simulink model "platooning_with_csma_simulink"  (R2017b)
settings: Solver=VariableStepAuto  StartTime=0.0  StopTime=t_end  FixedStep=timestep  RelTol=1e-3
model workspace (MAT data in the model file):
  t_0 = 0
values from neighbouring files (symbols this model uses):
  a_max = 1.0 * a_factor    (= 1)    [platooning_with_csma.m]
  a_min = -0.5 * a_factor    (= -0.5)    [platooning_with_csma.m]
  follower_1 = car    [platooning_with_csma.m]
  follower_2 = car    [platooning_with_csma.m]
  leader = car    [platooning_with_csma.m]
  N = 1000    [platooning_with_csma.m]
  remove_trigger_time = 0.01    [platooning_with_csma.m]
  timestep = 1e-3    (= 0.001)    [platooning_with_csma.m]
libraries: truetime x6, dspstat3 x2, dspindex x2, simulink x1
settings Model: Creator=s132652  LastModifiedBy=s132652
settings CodeAppCC: StateflowObjectComments=on

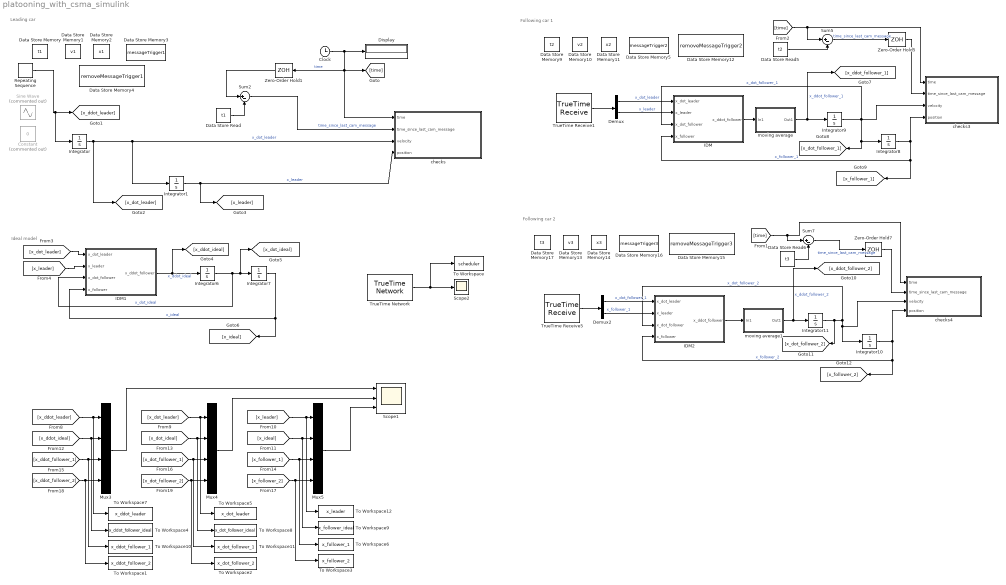
== system platooning_with_csma_simulink ==
  note: Leading car
  note: Ideal model
  note: Following car 1
  note: Following car 2
  Clock : Clock
  Constant : Constant  Commented=on  Value=0
  Data Store Memory : DataStoreMemory  DataStoreName=t1  ReadBeforeWriteMsg=warning  WriteAfterWriteMsg=warning  WriteAfterReadMsg=warning  ShowAdditionalParam=off
  Data Store Memory1 : DataStoreMemory  DataStoreName=v1  ReadBeforeWriteMsg=warning  WriteAfterWriteMsg=warning  WriteAfterReadMsg=warning  InitialValue=leader.v0  ShowAdditionalParam=off
  Data Store Memory10 : DataStoreMemory  DataStoreName=v2  ReadBeforeWriteMsg=warning  WriteAfterWriteMsg=warning  WriteAfterReadMsg=warning  InitialValue=follower_1.v0  ShowAdditionalParam=off
  Data Store Memory11 : DataStoreMemory  DataStoreName=x2  ReadBeforeWriteMsg=warning  WriteAfterWriteMsg=warning  WriteAfterReadMsg=warning  InitialValue=follower_1.x0  ShowAdditionalParam=off
  Data Store Memory12 : DataStoreMemory  DataStoreName=removeMessageTrigger2  ReadBeforeWriteMsg=warning  WriteAfterWriteMsg=warning  WriteAfterReadMsg=warning  ShowAdditionalParam=off
  Data Store Memory13 : DataStoreMemory  DataStoreName=v3  ReadBeforeWriteMsg=warning  WriteAfterWriteMsg=warning  WriteAfterReadMsg=warning  InitialValue=follower_2.v0  ShowAdditionalParam=off
  Data Store Memory14 : DataStoreMemory  DataStoreName=x3  ReadBeforeWriteMsg=warning  WriteAfterWriteMsg=warning  WriteAfterReadMsg=warning  InitialValue=follower_2.x0  ShowAdditionalParam=off
  Data Store Memory15 : DataStoreMemory  DataStoreName=removeMessageTrigger3  ReadBeforeWriteMsg=warning  WriteAfterWriteMsg=warning  WriteAfterReadMsg=warning  ShowAdditionalParam=off
  Data Store Memory16 : DataStoreMemory  DataStoreName=messageTrigger3  ReadBeforeWriteMsg=warning  WriteAfterWriteMsg=warning  WriteAfterReadMsg=warning  ShowAdditionalParam=off
  Data Store Memory17 : DataStoreMemory  DataStoreName=t3  ReadBeforeWriteMsg=warning  WriteAfterWriteMsg=warning  WriteAfterReadMsg=warning  ShowAdditionalParam=off
  Data Store Memory2 : DataStoreMemory  DataStoreName=x1  ReadBeforeWriteMsg=warning  WriteAfterWriteMsg=warning  WriteAfterReadMsg=warning  InitialValue=leader.x0  ShowAdditionalParam=off
  Data Store Memory3 : DataStoreMemory  DataStoreName=messageTrigger1  ReadBeforeWriteMsg=warning  WriteAfterWriteMsg=warning  WriteAfterReadMsg=warning  ShowAdditionalParam=off
  Data Store Memory4 : DataStoreMemory  DataStoreName=removeMessageTrigger1  ReadBeforeWriteMsg=warning  WriteAfterWriteMsg=warning  WriteAfterReadMsg=warning  ShowAdditionalParam=off
  Data Store Memory5 : DataStoreMemory  DataStoreName=messageTrigger2  ReadBeforeWriteMsg=warning  WriteAfterWriteMsg=warning  WriteAfterReadMsg=warning  ShowAdditionalParam=off
  Data Store Memory9 : DataStoreMemory  DataStoreName=t2  ReadBeforeWriteMsg=warning  WriteAfterWriteMsg=warning  WriteAfterReadMsg=warning  ShowAdditionalParam=off
  Data Store Read : DataStoreRead  DataStoreName=t1
  Data Store Read5 : DataStoreRead  DataStoreName=t2
  Data Store Read6 : DataStoreRead  DataStoreName=t3
  Demux : Demux  Outputs=2
  Demux2 : Demux  Outputs=2
  Display : Display
  IDM : Subsystem
  IDM1 : Subsystem
  IDM2 : Subsystem
  Integrator : Integrator  InitialCondition=leader.v0
  Integrator1 : Integrator  InitialCondition=leader.x0
  Integrator10 : Integrator  InitialCondition=follower_2.x0
  Integrator11 : Integrator  InitialCondition=follower_2.v0
  Integrator6 : Integrator  InitialCondition=follower_1.v0
  Integrator7 : Integrator  InitialCondition=follower_1.x0
  Integrator8 : Integrator  InitialCondition=follower_1.x0
  Integrator9 : Integrator  InitialCondition=follower_1.v0
  Mux3 : Mux
  Mux4 : Mux
  Mux5 : Mux
  Repeating Sequence : simulink/Sources/Repeating Sequence  rep_seq_t=[0 5 10 15 20 25 30 35 40 45 50 55 60 65 70]  rep_seq_y=[0 0 0 0 0 a_max a_max 0 0 0 a_min a_min 0 0 0]
  Scope1 : Scope  NumInputPorts=3
  Scope2 : Scope
  Sine Wave : Sin  Commented=on  Frequency=2*pi/10  SampleTime=0
  Sum2 : Sum  Inputs=|+-
  Sum5 : Sum  Inputs=|+-
  Sum7 : Sum  Inputs=|+-
  To Workspace : ToWorkspace  VariableName=scheduler  SaveFormat=Timeseries  SampleTime=-1
  To Workspace1 : ToWorkspace  VariableName=x_ddot_follower_2  SaveFormat=Timeseries  SampleTime=-1
  To Workspace10 : ToWorkspace  VariableName=x_ddot_follower_1  SaveFormat=Timeseries  SampleTime=-1
  To Workspace11 : ToWorkspace  VariableName=x_dot_follower_1  SaveFormat=Timeseries  SampleTime=-1
  To Workspace12 : ToWorkspace  VariableName=x_leader  SaveFormat=Timeseries  SampleTime=-1
  To Workspace2 : ToWorkspace  VariableName=x_dot_follower_2  SaveFormat=Timeseries  SampleTime=-1
  To Workspace3 : ToWorkspace  VariableName=x_follower_2  SaveFormat=Timeseries  SampleTime=-1
  To Workspace4 : ToWorkspace  VariableName=x_ddot_follower_ideal  SaveFormat=Timeseries  SampleTime=-1
  To Workspace5 : ToWorkspace  VariableName=x_dot_leader  SaveFormat=Timeseries  SampleTime=-1
  To Workspace6 : ToWorkspace  VariableName=x_follower_1  SaveFormat=Timeseries  SampleTime=-1
  To Workspace7 : ToWorkspace  VariableName=x_ddot_leader  SaveFormat=Timeseries  SampleTime=-1
  To Workspace8 : ToWorkspace  VariableName=x_dot_follower_ideal  SaveFormat=Timeseries  SampleTime=-1
  To Workspace9 : ToWorkspace  VariableName=x_follower_ideal  SaveFormat=Timeseries  SampleTime=-1
  TrueTime Network : truetime/TrueTime Network  nwtype=CSMA/AMP (CAN)  nwnbr=1  nnodes=3  rate=data_rate  minsize=512  lossprob=0  seed=0  bandwidths=[0.5 0.5]  slotsize=512  schedule=[1 1 2]  memsize=80000  buftype=Common buffer  overflow=Retransmit  dynSchedule=0  miniSlotSize=0  NIT=0  QSortMode=FIFO  sync=0  irtSchedule=0  nrtLength=0  nodeGraph=0  scheduleoutput=on
  TrueTime Receive1 : truetime/TrueTime Receive  nwnbr=1  receiver=1  outdim=2  triggeroutput=off  senderoutput=off  lengthoutput=off  priorityoutput=off  timestampoutput=off  signalpoweroutput=off  msgIDoutput=off
  TrueTime Receive5 : truetime/TrueTime Receive  nwnbr=1  receiver=2  outdim=2  triggeroutput=off  senderoutput=off  lengthoutput=off  priorityoutput=off  timestampoutput=off  signalpoweroutput=off  msgIDoutput=off
  Zero-Order Hold1 : ZeroOrderHold  SampleTime=timestep
  Zero-Order Hold5 : ZeroOrderHold  SampleTime=timestep
  Zero-Order Hold7 : ZeroOrderHold  SampleTime=timestep
  checks : Subsystem
  checks3 : Subsystem
  checks4 : Subsystem
  moving average : Subsystem
  moving average1 : Subsystem
  wires:
  TrueTime Network/1 -> To Workspace/1, Scope2/1
  Sum2/1 -> checks/2(time_since_last_cam_message)  "time_since_last_cam_message"
  Data Store Read/1 -> Sum2/2
  Integrator6/1 -> IDM1/3(x_dot_follower), [x_dot_ideal], Integrator7/1  "x_dot_ideal"
  Integrator/1 -> [x_dot_leader], Integrator1/1, checks/3(velocity)  "x_dot_leader"
  IDM1/1(x_ddot_follower) -> [x_ddot_ideal], Integrator6/1  "x_ddot_ideal"
  Integrator7/1 -> [x_ideal], IDM1/4(x_follower)  "x_ideal"
  Integrator1/1 -> [x_leader], checks/4(position)  "x_leader"
  moving average/1(Out1) -> [x_ddot_follower_1], Integrator9/1  "x_ddot_follower_1"
  Integrator8/1 -> [x_follower_1], IDM/4(x_follower), checks3/4(position)  "x_follower_1"
  Integrator9/1 -> [x_dot_follower_1], Integrator8/1, checks3/3(velocity), IDM/3(x_dot_follower)  "x_dot_follower_1"
  IDM/1(x_ddot_follower) -> moving average/1(In1)
  TrueTime Receive1/1 -> Demux/1
  Zero-Order Hold5/1 -> checks3/2(time_since_last_cam_message)
  Data Store Read5/1 -> Sum5/2
  Sum5/1 -> Zero-Order Hold5/1  "time_since_last_cam_message"
  Clock/1 -> checks/1(time), [time], Zero-Order Hold1/1, Display/1  "time"
  Zero-Order Hold7/1 -> checks4/2(time_since_last_cam_message)
  moving average1/1(Out1) -> [x_ddot_follower_2], Integrator11/1  "x_ddot_follower_2"
  Sum7/1 -> Zero-Order Hold7/1  "time_since_last_cam_message"
  TrueTime Receive5/1 -> Demux2/1
  Data Store Read6/1 -> Sum7/2
  Integrator10/1 -> IDM2/4(x_follower), [x_follower_2], checks4/4(position)  "x_follower_2"
  Integrator11/1 -> [x_dot_follower_2], IDM2/3(x_dot_follower), checks4/3(velocity), Integrator10/1  "x_dot_follower_2"
  IDM2/1(x_ddot_follower) -> moving average1/1(In1)
  [time] -> checks4/1(time), Sum7/1
  [time] -> Sum5/1, checks3/1(time)
  [x_dot_leader] -> IDM1/1(x_dot_leader)
  [x_leader] -> IDM1/2(x_leader)
  [x_ddot_leader] -> To Workspace7/1, Mux3/1
  [x_ddot_ideal] -> To Workspace4/1, Mux3/2
  [x_ddot_follower_1] -> To Workspace10/1, Mux3/3
  [x_ddot_follower_2] -> To Workspace1/1, Mux3/4
  [x_dot_leader] -> To Workspace5/1, Mux4/1
  [x_dot_ideal] -> To Workspace8/1, Mux4/2
  [x_dot_follower_1] -> To Workspace11/1, Mux4/3
  [x_dot_follower_2] -> To Workspace2/1, Mux4/4
  [x_follower_2] -> To Workspace3/1, Mux5/4
  [x_follower_1] -> To Workspace6/1, Mux5/3
  [x_ideal] -> To Workspace9/1, Mux5/2
  [x_leader] -> To Workspace12/1, Mux5/1
  Mux3/1 -> Scope1/1
  Mux4/1 -> Scope1/2
  Mux5/1 -> Scope1/3
  Zero-Order Hold1/1 -> Sum2/1
  Demux/2 -> IDM/2(x_leader)  "x_leader"
  Demux/1 -> IDM/1(x_dot_leader)  "x_dot_leader"
  Demux2/1 -> IDM2/1(x_dot_leader)  "x_dot_follower_1"
  Demux2/2 -> IDM2/2(x_leader)  "x_follower_1"
  Repeating Sequence/1 -> Integrator/1, [x_ddot_leader]

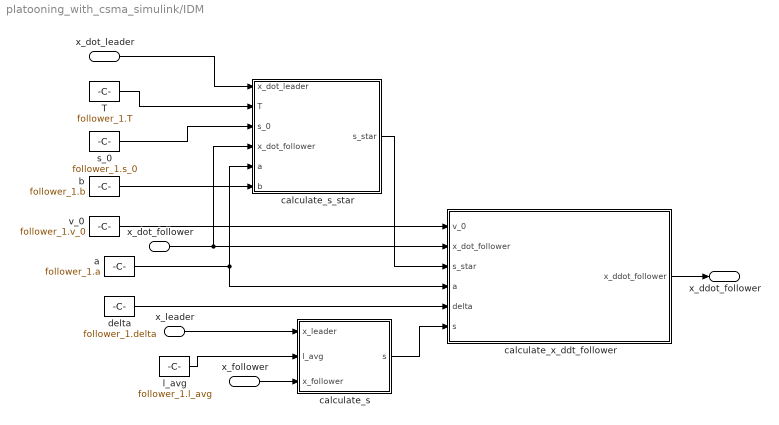
== system platooning_with_csma_simulink/IDM ==
  x_dot_leader : Inport
  x_leader : Inport  Port=2
  x_dot_follower : Inport  Port=3
  x_follower : Inport  Port=4
  T : Constant  Value=follower_1.T
  a : Constant  Value=follower_1.a
  b : Constant  Value=follower_1.b
  calculate_s : Subsystem
  calculate_s_star : Subsystem
  calculate_x_ddt_follower : Subsystem
  delta : Constant  Value=follower_1.delta
  l_avg : Constant  Value=follower_1.l_avg
  s_0 : Constant  Value=follower_1.s_0
  v_0 : Constant  Value=follower_1.v_0
  x_ddot_follower : Outport
  wires:
  v_0/1 -> calculate_x_ddt_follower/1(v_0)
  T/1 -> calculate_s_star/2(T)
  s_0/1 -> calculate_s_star/3(s_0)
  calculate_x_ddt_follower/1(x_ddot_follower) -> x_ddot_follower/1
  b/1 -> calculate_s_star/6(b)
  l_avg/1 -> calculate_s/2(l_avg)
  calculate_s/1(s) -> calculate_x_ddt_follower/6(s)
  delta/1 -> calculate_x_ddt_follower/5(delta)
  calculate_s_star/1(s_star) -> calculate_x_ddt_follower/3(s_star)
  x_follower/1 -> calculate_s/3(x_follower)
  x_dot_leader/1 -> calculate_s_star/1(x_dot_leader)
  x_leader/1 -> calculate_s/1(x_leader)
  x_dot_follower/1 -> calculate_s_star/4(x_dot_follower), calculate_x_ddt_follower/2(x_dot_follower)
  a/1 -> calculate_x_ddt_follower/4(a), calculate_s_star/5(a)

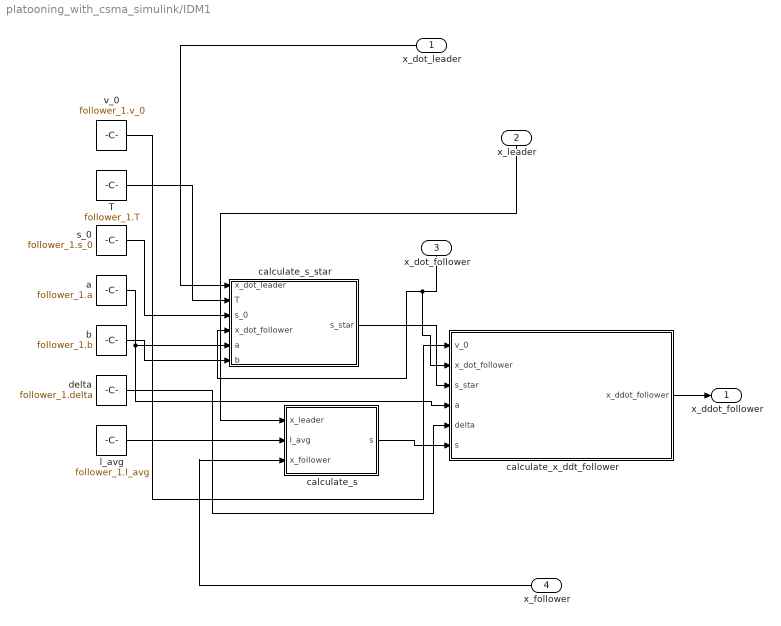
== system platooning_with_csma_simulink/IDM1 ==
  x_dot_leader : Inport
  x_leader : Inport  Port=2
  x_dot_follower : Inport  Port=3
  x_follower : Inport  Port=4
  T : Constant  Value=follower_1.T
  a : Constant  Value=follower_1.a
  b : Constant  Value=follower_1.b
  calculate_s : Subsystem
  calculate_s_star : Subsystem
  calculate_x_ddt_follower : Subsystem
  delta : Constant  Value=follower_1.delta
  l_avg : Constant  Value=follower_1.l_avg
  "s_0 " : Constant  Value=follower_1.s_0
  v_0 : Constant  Value=follower_1.v_0
  x_ddot_follower : Outport
  wires:
  a/1 -> calculate_x_ddt_follower/4(a), calculate_s_star/5(a)
  v_0/1 -> calculate_x_ddt_follower/1(v_0)
  T/1 -> calculate_s_star/2(T)
  "s_0 "/1 -> calculate_s_star/3(s_0)
  calculate_x_ddt_follower/1(x_ddot_follower) -> x_ddot_follower/1
  b/1 -> calculate_s_star/6(b)
  l_avg/1 -> calculate_s/2(l_avg)
  calculate_s/1(s) -> calculate_x_ddt_follower/6(s)
  delta/1 -> calculate_x_ddt_follower/5(delta)
  calculate_s_star/1(s_star) -> calculate_x_ddt_follower/3(s_star)
  x_follower/1 -> calculate_s/3(x_follower)
  x_dot_follower/1 -> calculate_x_ddt_follower/2(x_dot_follower), calculate_s_star/4(x_dot_follower)
  x_dot_leader/1 -> calculate_s_star/1(x_dot_leader)
  x_leader/1 -> calculate_s/1(x_leader)

== system platooning_with_csma_simulink/IDM2 ==
  x_dot_leader : Inport
  x_leader : Inport  Port=2
  x_dot_follower : Inport  Port=3
  x_follower : Inport  Port=4
  T : Constant  Value=follower_2.T
  a : Constant  Value=follower_2.a
  b : Constant  Value=follower_2.b
  calculate_s : Subsystem
  calculate_s_star : Subsystem
  calculate_x_ddt_follower : Subsystem
  delta : Constant  Value=follower_2.delta
  l_avg : Constant  Value=follower_2.l_avg
  s_0 : Constant  Value=follower_2.s_0
  v_0 : Constant  Value=follower_2.v_0
  x_ddot_follower : Outport
  wires:
  v_0/1 -> calculate_x_ddt_follower/1(v_0)
  T/1 -> calculate_s_star/2(T)
  s_0/1 -> calculate_s_star/3(s_0)
  calculate_x_ddt_follower/1(x_ddot_follower) -> x_ddot_follower/1
  b/1 -> calculate_s_star/6(b)
  l_avg/1 -> calculate_s/2(l_avg)
  calculate_s/1(s) -> calculate_x_ddt_follower/6(s)
  delta/1 -> calculate_x_ddt_follower/5(delta)
  calculate_s_star/1(s_star) -> calculate_x_ddt_follower/3(s_star)
  x_follower/1 -> calculate_s/3(x_follower)
  x_dot_leader/1 -> calculate_s_star/1(x_dot_leader)
  x_leader/1 -> calculate_s/1(x_leader)
  x_dot_follower/1 -> calculate_s_star/4(x_dot_follower), calculate_x_ddt_follower/2(x_dot_follower)
  a/1 -> calculate_x_ddt_follower/4(a), calculate_s_star/5(a)

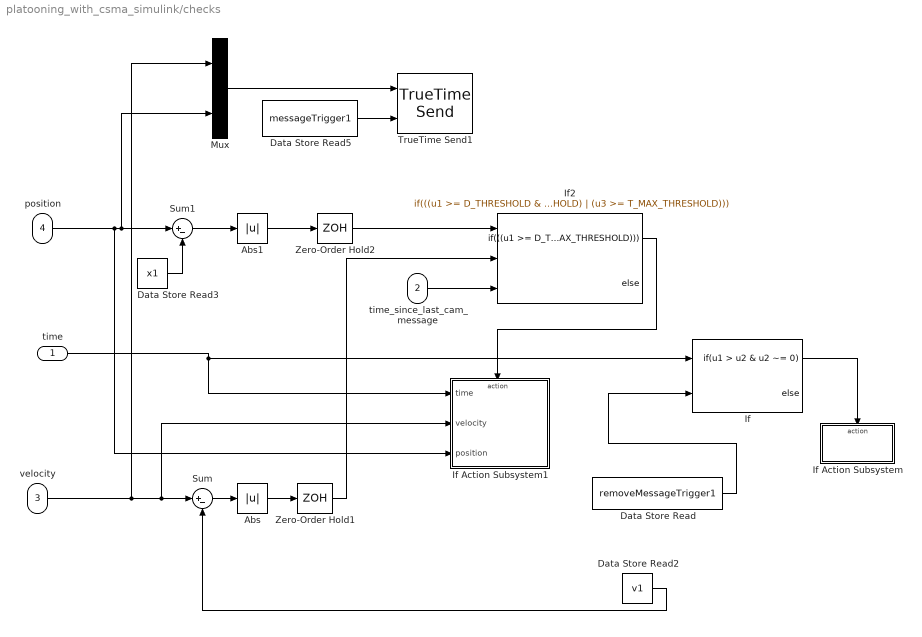
== system platooning_with_csma_simulink/checks ==
  time : Inport
  time_since_last_cam_message : Inport  Port=2
  velocity : Inport  Port=3
  position : Inport  Port=4
  Abs : Abs
  Abs1 : Abs
  Data Store Read : DataStoreRead  DataStoreName=removeMessageTrigger1
  Data Store Read2 : DataStoreRead  DataStoreName=v1
  Data Store Read3 : DataStoreRead  DataStoreName=x1
  Data Store Read5 : DataStoreRead  DataStoreName=messageTrigger1
  If : If  NumInputs=2  IfExpression=u1 > u2 & u2 ~= 0
  If Action Subsystem : Subsystem  TreatAsAtomicUnit=on
  If Action Subsystem1 : Subsystem  TreatAsAtomicUnit=on
  If2 : If  NumInputs=3  IfExpression=((u1 >= D_THRESHOLD & u3 >= T_MIN_THRESHOLD) | (u2 >= S_THRESHOLD & u3 >= T_MIN_THRESHOLD) | (u3 >= T_MAX_THRESHOLD))
  Mux : Mux  Inputs=2
  Sum : Sum  Inputs=|+-
  Sum1 : Sum  Inputs=|+-
  TrueTime Send1 : truetime/TrueTime Send  trigger=rising  nwnbr=1  sender=1  indim=2  recsource=internal  receiver=1  lengthsource=internal  length=data_length  priosource=internal  prio=1  msgIDsource=internal  msgID=0  dynamicSegment=dynamic
  Zero-Order Hold1 : ZeroOrderHold  SampleTime=timestep
  Zero-Order Hold2 : ZeroOrderHold  SampleTime=timestep
  wires:
  Data Store Read3/1 -> Sum1/2
  Sum1/1 -> Abs1/1
  Abs1/1 -> Zero-Order Hold2/1
  Zero-Order Hold2/1 -> If2/1
  time/1 -> If/1, If Action Subsystem1/1(time)
  position/1 -> Mux/2, Sum1/1, If Action Subsystem1/3(position)
  If2/1 -> If Action Subsystem1/Action
  Abs/1 -> Zero-Order Hold1/1
  Sum/1 -> Abs/1
  Data Store Read2/1 -> Sum/2
  velocity/1 -> Mux/1, If Action Subsystem1/2(velocity), Sum/1
  time_since_last_cam_message/1 -> If2/3
  Zero-Order Hold1/1 -> If2/2
  Mux/1 -> TrueTime Send1/1
  Data Store Read5/1 -> TrueTime Send1/2
  If/1 -> If Action Subsystem/Action
  Data Store Read/1 -> If/2

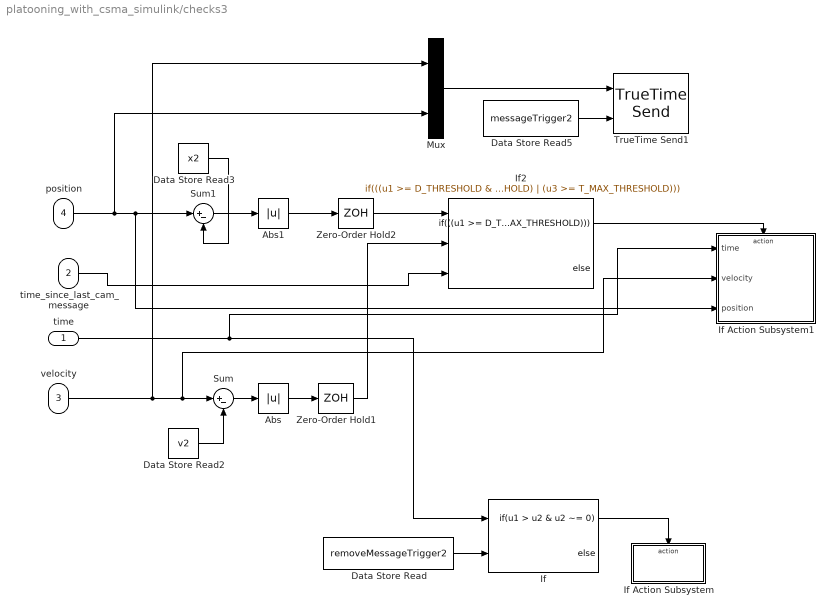
== system platooning_with_csma_simulink/checks3 ==
  time : Inport
  time_since_last_cam_message : Inport  Port=2
  velocity : Inport  Port=3
  position : Inport  Port=4
  Abs : Abs
  Abs1 : Abs
  Data Store Read : DataStoreRead  DataStoreName=removeMessageTrigger2
  Data Store Read2 : DataStoreRead  DataStoreName=v2
  Data Store Read3 : DataStoreRead  DataStoreName=x2
  Data Store Read5 : DataStoreRead  DataStoreName=messageTrigger2
  If : If  NumInputs=2  IfExpression=u1 > u2 & u2 ~= 0
  If Action Subsystem : Subsystem  TreatAsAtomicUnit=on
  If Action Subsystem1 : Subsystem  TreatAsAtomicUnit=on
  If2 : If  NumInputs=3  IfExpression=((u1 >= D_THRESHOLD & u3 >= T_MIN_THRESHOLD) | (u2 >= S_THRESHOLD & u3 >= T_MIN_THRESHOLD) | (u3 >= T_MAX_THRESHOLD))
  Mux : Mux  Inputs=2
  Sum : Sum  Inputs=|+-
  Sum1 : Sum  Inputs=|+-
  TrueTime Send1 : truetime/TrueTime Send  trigger=rising  nwnbr=1  sender=2  indim=2  recsource=internal  receiver=2  lengthsource=internal  length=data_length  priosource=internal  prio=1  msgIDsource=internal  msgID=0  dynamicSegment=dynamic
  Zero-Order Hold1 : ZeroOrderHold  SampleTime=timestep
  Zero-Order Hold2 : ZeroOrderHold  SampleTime=timestep
  wires:
  Data Store Read3/1 -> Sum1/2
  Sum1/1 -> Abs1/1
  Abs1/1 -> Zero-Order Hold2/1
  Zero-Order Hold2/1 -> If2/1
  time/1 -> If/1, If Action Subsystem1/1(time)
  position/1 -> Mux/2, If Action Subsystem1/3(position), Sum1/1
  If2/1 -> If Action Subsystem1/Action
  Abs/1 -> Zero-Order Hold1/1
  Sum/1 -> Abs/1
  Data Store Read2/1 -> Sum/2
  velocity/1 -> If Action Subsystem1/2(velocity), Sum/1, Mux/1
  time_since_last_cam_message/1 -> If2/3
  Zero-Order Hold1/1 -> If2/2
  Mux/1 -> TrueTime Send1/1
  Data Store Read5/1 -> TrueTime Send1/2
  If/1 -> If Action Subsystem/Action
  Data Store Read/1 -> If/2

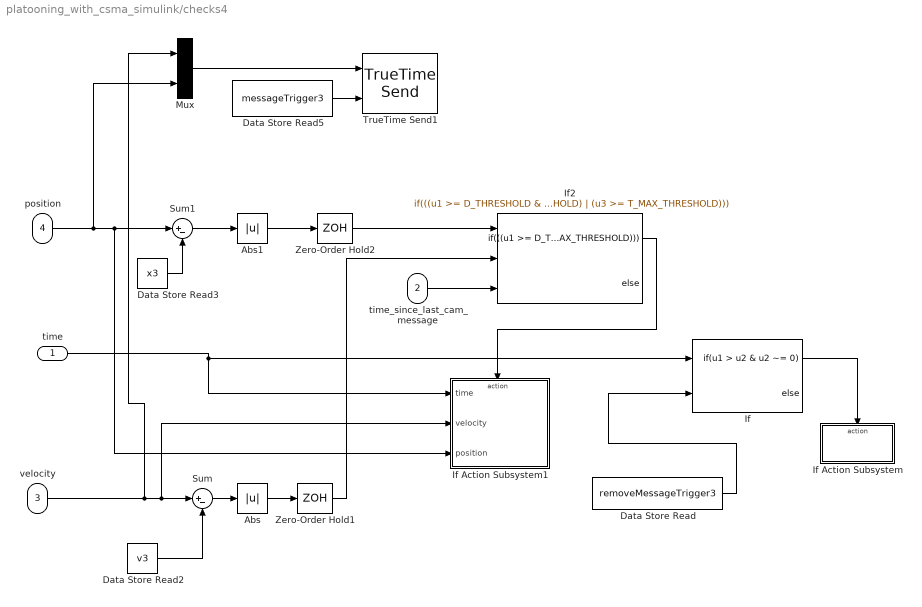
== system platooning_with_csma_simulink/checks4 ==
  time : Inport
  time_since_last_cam_message : Inport  Port=2
  velocity : Inport  Port=3
  position : Inport  Port=4
  Abs : Abs
  Abs1 : Abs
  Data Store Read : DataStoreRead  DataStoreName=removeMessageTrigger3
  Data Store Read2 : DataStoreRead  DataStoreName=v3
  Data Store Read3 : DataStoreRead  DataStoreName=x3
  Data Store Read5 : DataStoreRead  DataStoreName=messageTrigger3
  If : If  NumInputs=2  IfExpression=u1 > u2 & u2 ~= 0
  If Action Subsystem : Subsystem  TreatAsAtomicUnit=on
  If Action Subsystem1 : Subsystem  TreatAsAtomicUnit=on
  If2 : If  NumInputs=3  IfExpression=((u1 >= D_THRESHOLD & u3 >= T_MIN_THRESHOLD) | (u2 >= S_THRESHOLD & u3 >= T_MIN_THRESHOLD) | (u3 >= T_MAX_THRESHOLD))
  Mux : Mux  Inputs=2
  Sum : Sum  Inputs=|+-
  Sum1 : Sum  Inputs=|+-
  TrueTime Send1 : truetime/TrueTime Send  trigger=rising  nwnbr=1  sender=3  indim=2  recsource=internal  receiver=3  lengthsource=internal  length=data_length  priosource=internal  prio=1  msgIDsource=internal  msgID=0  dynamicSegment=dynamic
  Zero-Order Hold1 : ZeroOrderHold  SampleTime=-1
  Zero-Order Hold2 : ZeroOrderHold  SampleTime=timestep
  wires:
  Data Store Read3/1 -> Sum1/2
  Sum1/1 -> Abs1/1
  Abs1/1 -> Zero-Order Hold2/1
  Zero-Order Hold2/1 -> If2/1
  time/1 -> If/1, If Action Subsystem1/1(time)
  position/1 -> Mux/2, Sum1/1, If Action Subsystem1/3(position)
  If2/1 -> If Action Subsystem1/Action
  Abs/1 -> Zero-Order Hold1/1
  Sum/1 -> Abs/1
  Data Store Read2/1 -> Sum/2
  velocity/1 -> Mux/1, If Action Subsystem1/2(velocity), Sum/1
  time_since_last_cam_message/1 -> If2/3
  Zero-Order Hold1/1 -> If2/2
  Mux/1 -> TrueTime Send1/1
  Data Store Read5/1 -> TrueTime Send1/2
  If/1 -> If Action Subsystem/Action
  Data Store Read/1 -> If/2

== system platooning_with_csma_simulink/moving average ==
  note: moving average
  In1 : Inport
  IC : InitialCondition  Value=zeros(N,1)
  Mean : dspstat3/Mean  run=off  reset_popup=None  InputProcessing=Columns as channels (frame based)  directionMode=Each column  dimension=1  roiEnable=off  roiType=Rectangles  roiPortion=Entire ROI  roiOutput=Individual statistics for each ROI  roiFlag=off  outputDataTypeStr=Inherit: Same as accumulator  outputLastDataTypeStr=Inherit: Same as accumulator  outputMin=[]  outputMax=[]  roundingMode=Floor  overflowMode=off
  Memory : Memory
  Mux : Mux  Inputs=2
  Variable Selector : dspindex/Variable Selector  NumInputs=1  rowsOrCols=Rows  IdxMode=Fixed  Elements=1:N-1  ZerOneIdxMode=One-based  errmode=Clip Index  FillMode=on  FillValues=0
  Out1 : Outport
  wires:
  In1/1 -> Mux/1
  Mux/1 -> Mean/1, Memory/1
  Memory/1 -> IC/1
  IC/1 -> Variable Selector/1
  Mean/1 -> Out1/1
  Variable Selector/1 -> Mux/2

== system platooning_with_csma_simulink/moving average1 ==
  note: moving average
  In1 : Inport
  IC : InitialCondition  Value=zeros(N,1)
  Mean : dspstat3/Mean  run=off  reset_popup=None  InputProcessing=Columns as channels (frame based)  directionMode=Each column  dimension=1  roiEnable=off  roiType=Rectangles  roiPortion=Entire ROI  roiOutput=Individual statistics for each ROI  roiFlag=off  outputDataTypeStr=Inherit: Same as accumulator  outputLastDataTypeStr=Inherit: Same as accumulator  outputMin=[]  outputMax=[]  roundingMode=Floor  overflowMode=off
  Memory : Memory
  Mux : Mux  Inputs=2
  Variable Selector : dspindex/Variable Selector  NumInputs=1  rowsOrCols=Rows  IdxMode=Fixed  Elements=1:N-1  ZerOneIdxMode=One-based  errmode=Clip Index  FillMode=on  FillValues=0
  Out1 : Outport
  wires:
  In1/1 -> Mux/1
  Mux/1 -> Mean/1, Memory/1
  Memory/1 -> IC/1
  IC/1 -> Variable Selector/1
  Mean/1 -> Out1/1
  Variable Selector/1 -> Mux/2

== system platooning_with_csma_simulink/IDM/calculate_s ==
  x_leader : Inport
  l_avg : Inport  Port=2
  x_follower : Inport  Port=3
  Sum3 : Sum  Inputs=|+-
  Sum4 : Sum  Inputs=|+-
  s : Outport
  wires:
  Sum4/1 -> s/1  "s"
  Sum3/1 -> Sum4/1
  l_avg/1 -> Sum4/2
  x_follower/1 -> Sum3/2
  x_leader/1 -> Sum3/1

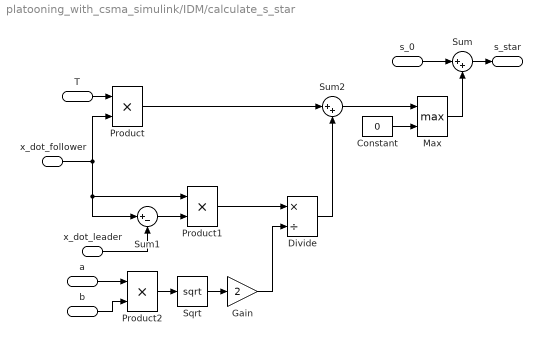
== system platooning_with_csma_simulink/IDM/calculate_s_star ==
  x_dot_leader : Inport
  T : Inport  Port=2
  s_0 : Inport  Port=3
  x_dot_follower : Inport  Port=4
  a : Inport  Port=5
  b : Inport  Port=6
  Constant : Constant  Value=0
  Divide : Product  Inputs=*/
  Gain : Gain  Gain=2
  Max : MinMax  Function=max  Inputs=2
  Product : Product
  Product1 : Product
  Product2 : Product
  Sqrt : Sqrt  SaturateOnIntegerOverflow=on
  Sum : Sum  Inputs=|++
  Sum1 : Sum  Inputs=|+-
  Sum2 : Sum  Inputs=|++
  s_star : Outport
  wires:
  Sum1/1 -> Product1/2
  T/1 -> Product/1
  s_0/1 -> Sum/1
  Product1/1 -> Divide/1
  Product/1 -> Sum2/1
  Divide/1 -> Sum2/2
  x_dot_leader/1 -> Sum1/2
  Product2/1 -> Sqrt/1
  Sqrt/1 -> Gain/1
  Gain/1 -> Divide/2
  a/1 -> Product2/1
  b/1 -> Product2/2
  Constant/1 -> Max/2
  Sum2/1 -> Max/1
  Max/1 -> Sum/2
  Sum/1 -> s_star/1
  x_dot_follower/1 -> Product/2, Product1/1, Sum1/1

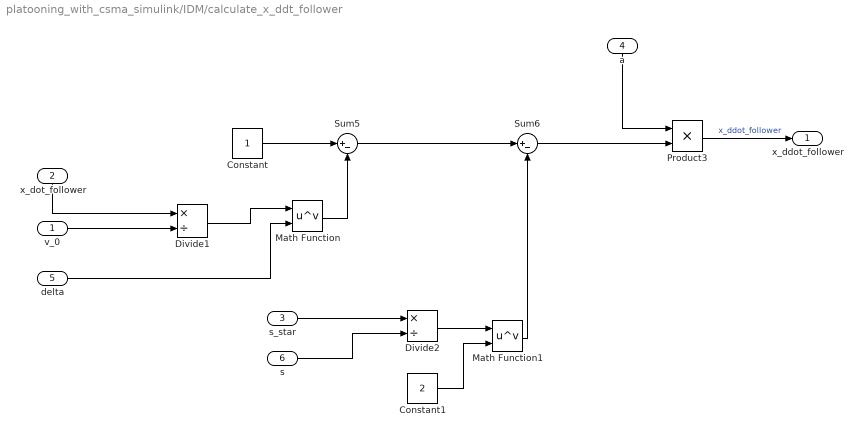
== system platooning_with_csma_simulink/IDM/calculate_x_ddt_follower ==
  v_0 : Inport
  x_dot_follower : Inport  Port=2
  s_star : Inport  Port=3
  a : Inport  Port=4
  delta : Inport  Port=5
  s : Inport  Port=6
  Constant : Constant
  Constant1 : Constant  Value=2
  Divide1 : Product  Inputs=*/
  Divide2 : Product  Inputs=*/
  Math Function : Math  Operator=pow  SaturateOnIntegerOverflow=on
  Math Function1 : Math  Operator=pow  SaturateOnIntegerOverflow=on
  Product3 : Product
  Sum5 : Sum  Inputs=|+-
  Sum6 : Sum  Inputs=|+-
  x_ddot_follower : Outport
  wires:
  Product3/1 -> x_ddot_follower/1  "x_ddot_follower"
  v_0/1 -> Divide1/2
  Constant/1 -> Sum5/1
  Math Function/1 -> Sum5/2
  a/1 -> Product3/1
  x_dot_follower/1 -> Divide1/1
  s/1 -> Divide2/2
  s_star/1 -> Divide2/1
  Sum5/1 -> Sum6/1
  Constant1/1 -> Math Function1/2
  Divide1/1 -> Math Function/1
  Math Function1/1 -> Sum6/2
  delta/1 -> Math Function/2
  Divide2/1 -> Math Function1/1
  Sum6/1 -> Product3/2

== system platooning_with_csma_simulink/IDM1/calculate_s ==
  x_leader : Inport
  l_avg : Inport  Port=2
  x_follower : Inport  Port=3
  Sum3 : Sum  Inputs=|+-
  Sum4 : Sum  Inputs=|+-
  s : Outport
  wires:
  Sum4/1 -> s/1  "s"
  Sum3/1 -> Sum4/1
  l_avg/1 -> Sum4/2
  x_follower/1 -> Sum3/2
  x_leader/1 -> Sum3/1

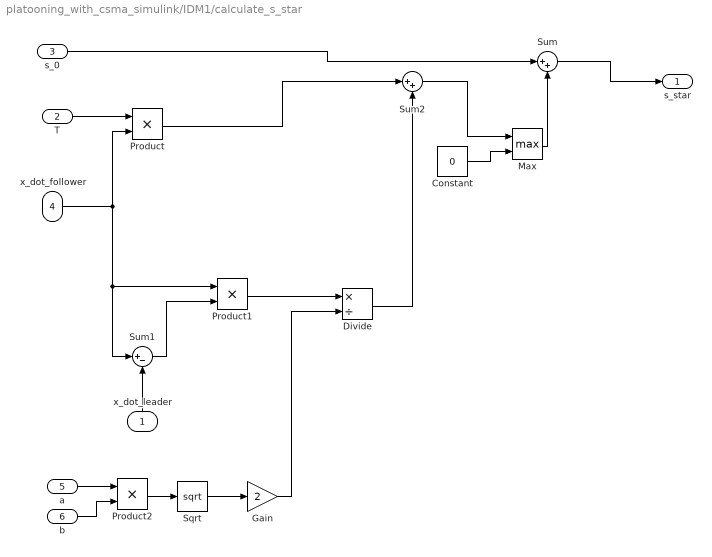
== system platooning_with_csma_simulink/IDM1/calculate_s_star ==
  x_dot_leader : Inport
  T : Inport  Port=2
  s_0 : Inport  Port=3
  x_dot_follower : Inport  Port=4
  a : Inport  Port=5
  b : Inport  Port=6
  Constant : Constant  Value=0
  Divide : Product  Inputs=*/
  Gain : Gain  Gain=2
  Max : MinMax  Function=max  Inputs=2
  Product : Product
  Product1 : Product
  Product2 : Product
  Sqrt : Sqrt  SaturateOnIntegerOverflow=on
  Sum : Sum  Inputs=|++
  Sum1 : Sum  Inputs=|+-
  Sum2 : Sum  Inputs=|++
  s_star : Outport
  wires:
  Sum1/1 -> Product1/2
  T/1 -> Product/1
  s_0/1 -> Sum/1
  Product1/1 -> Divide/1
  Product/1 -> Sum2/1
  Divide/1 -> Sum2/2
  x_dot_leader/1 -> Sum1/2
  x_dot_follower/1 -> Product/2, Sum1/1, Product1/1
  Product2/1 -> Sqrt/1
  Sqrt/1 -> Gain/1
  Gain/1 -> Divide/2
  a/1 -> Product2/1
  b/1 -> Product2/2
  Constant/1 -> Max/2
  Sum2/1 -> Max/1
  Max/1 -> Sum/2
  Sum/1 -> s_star/1

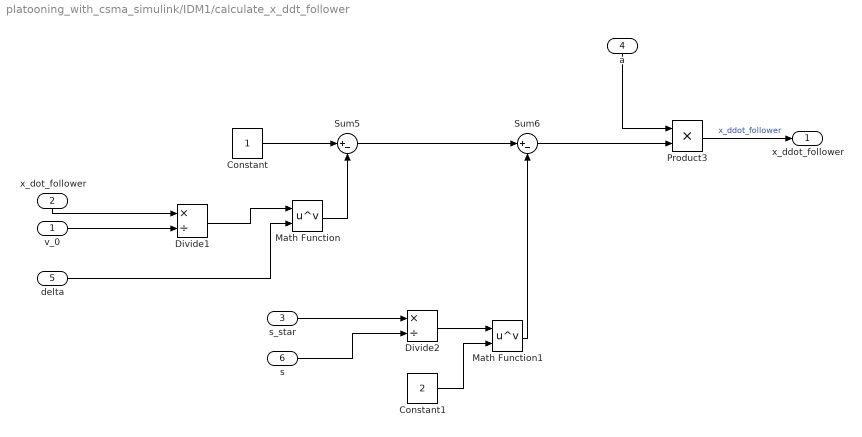
== system platooning_with_csma_simulink/IDM1/calculate_x_ddt_follower ==
  v_0 : Inport
  x_dot_follower : Inport  Port=2
  s_star : Inport  Port=3
  a : Inport  Port=4
  delta : Inport  Port=5
  s : Inport  Port=6
  Constant : Constant
  Constant1 : Constant  Value=2
  Divide1 : Product  Inputs=*/
  Divide2 : Product  Inputs=*/
  Math Function : Math  Operator=pow  SaturateOnIntegerOverflow=on
  Math Function1 : Math  Operator=pow  SaturateOnIntegerOverflow=on
  Product3 : Product
  Sum5 : Sum  Inputs=|+-
  Sum6 : Sum  Inputs=|+-
  x_ddot_follower : Outport
  wires:
  Product3/1 -> x_ddot_follower/1  "x_ddot_follower"
  v_0/1 -> Divide1/2
  Constant/1 -> Sum5/1
  Math Function/1 -> Sum5/2
  a/1 -> Product3/1
  x_dot_follower/1 -> Divide1/1
  s/1 -> Divide2/2
  s_star/1 -> Divide2/1
  Sum5/1 -> Sum6/1
  Constant1/1 -> Math Function1/2
  Divide1/1 -> Math Function/1
  Math Function1/1 -> Sum6/2
  delta/1 -> Math Function/2
  Divide2/1 -> Math Function1/1
  Sum6/1 -> Product3/2

== system platooning_with_csma_simulink/IDM2/calculate_s ==
  x_leader : Inport
  l_avg : Inport  Port=2
  x_follower : Inport  Port=3
  Sum3 : Sum  Inputs=|+-
  Sum4 : Sum  Inputs=|+-
  s : Outport
  wires:
  Sum4/1 -> s/1  "s"
  Sum3/1 -> Sum4/1
  l_avg/1 -> Sum4/2
  x_follower/1 -> Sum3/2
  x_leader/1 -> Sum3/1

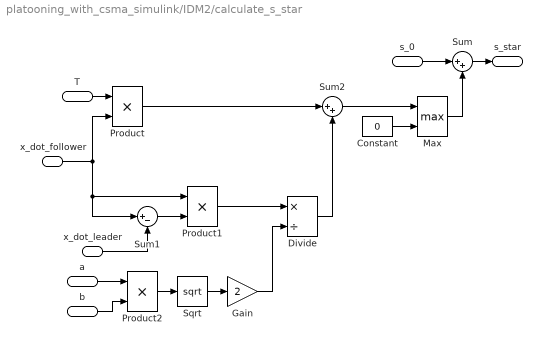
== system platooning_with_csma_simulink/IDM2/calculate_s_star ==
  x_dot_leader : Inport
  T : Inport  Port=2
  s_0 : Inport  Port=3
  x_dot_follower : Inport  Port=4
  a : Inport  Port=5
  b : Inport  Port=6
  Constant : Constant  Value=0
  Divide : Product  Inputs=*/
  Gain : Gain  Gain=2
  Max : MinMax  Function=max  Inputs=2
  Product : Product
  Product1 : Product
  Product2 : Product
  Sqrt : Sqrt  SaturateOnIntegerOverflow=on
  Sum : Sum  Inputs=|++
  Sum1 : Sum  Inputs=|+-
  Sum2 : Sum  Inputs=|++
  s_star : Outport
  wires:
  Sum1/1 -> Product1/2
  T/1 -> Product/1
  s_0/1 -> Sum/1
  Product1/1 -> Divide/1
  Product/1 -> Sum2/1
  Divide/1 -> Sum2/2
  x_dot_leader/1 -> Sum1/2
  Product2/1 -> Sqrt/1
  Sqrt/1 -> Gain/1
  Gain/1 -> Divide/2
  a/1 -> Product2/1
  b/1 -> Product2/2
  Constant/1 -> Max/2
  Sum2/1 -> Max/1
  Max/1 -> Sum/2
  Sum/1 -> s_star/1
  x_dot_follower/1 -> Product/2, Product1/1, Sum1/1

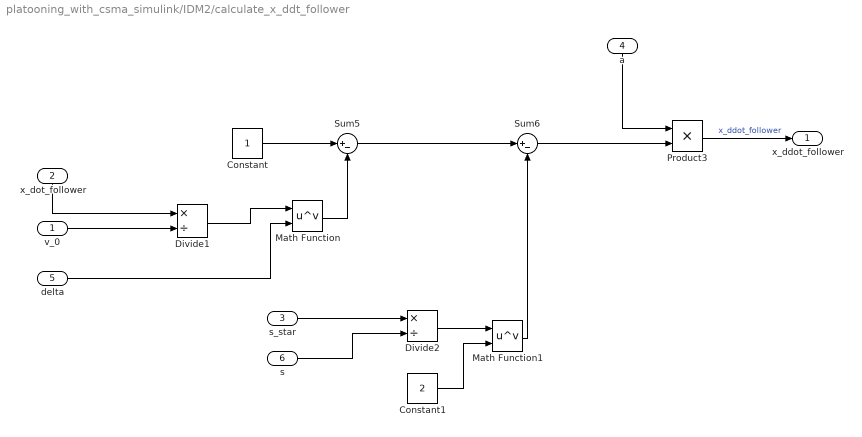
== system platooning_with_csma_simulink/IDM2/calculate_x_ddt_follower ==
  v_0 : Inport
  x_dot_follower : Inport  Port=2
  s_star : Inport  Port=3
  a : Inport  Port=4
  delta : Inport  Port=5
  s : Inport  Port=6
  Constant : Constant
  Constant1 : Constant  Value=2
  Divide1 : Product  Inputs=*/
  Divide2 : Product  Inputs=*/
  Math Function : Math  Operator=pow  SaturateOnIntegerOverflow=on
  Math Function1 : Math  Operator=pow  SaturateOnIntegerOverflow=on
  Product3 : Product
  Sum5 : Sum  Inputs=|+-
  Sum6 : Sum  Inputs=|+-
  x_ddot_follower : Outport
  wires:
  Product3/1 -> x_ddot_follower/1  "x_ddot_follower"
  v_0/1 -> Divide1/2
  Constant/1 -> Sum5/1
  Math Function/1 -> Sum5/2
  a/1 -> Product3/1
  x_dot_follower/1 -> Divide1/1
  s/1 -> Divide2/2
  s_star/1 -> Divide2/1
  Sum5/1 -> Sum6/1
  Constant1/1 -> Math Function1/2
  Divide1/1 -> Math Function/1
  Math Function1/1 -> Sum6/2
  delta/1 -> Math Function/2
  Divide2/1 -> Math Function1/1
  Sum6/1 -> Product3/2

== system platooning_with_csma_simulink/checks/If Action Subsystem ==
  Action Port : ActionPort  ActionType=then
  Constant : Constant  Value=0
  Constant1 : Constant  Value=0
  Data Store Write : DataStoreWrite  DataStoreName=messageTrigger1
  Data Store Write4 : DataStoreWrite  DataStoreName=removeMessageTrigger1
  wires:
  Constant/1 -> Data Store Write4/1
  Constant1/1 -> Data Store Write/1

== system platooning_with_csma_simulink/checks/If Action Subsystem1 ==
  time : Inport
  velocity : Inport  Port=2
  position : Inport  Port=3
  Action Port : ActionPort  ActionType=then
  Constant : Constant
  Constant1 : Constant  Value=remove_trigger_time
  Data Store Read3 : DataStoreRead  DataStoreName=messageTrigger1
  Data Store Write : DataStoreWrite  DataStoreName=t1
  Data Store Write1 : DataStoreWrite  DataStoreName=messageTrigger1
  Data Store Write2 : DataStoreWrite  DataStoreName=v1
  Data Store Write3 : DataStoreWrite  DataStoreName=x1
  Data Store Write4 : DataStoreWrite  DataStoreName=removeMessageTrigger1
  Sum : Sum  Inputs=|++
  Sum1 : Sum  Inputs=|++
  wires:
  time/1 -> Sum1/1, Data Store Write/1
  position/1 -> Data Store Write3/1
  velocity/1 -> Data Store Write2/1
  Data Store Read3/1 -> Sum/1
  Constant/1 -> Sum/2
  Sum/1 -> Data Store Write1/1
  Sum1/1 -> Data Store Write4/1
  Constant1/1 -> Sum1/2

== system platooning_with_csma_simulink/checks3/If Action Subsystem ==
  Action Port : ActionPort  ActionType=then
  Constant : Constant  Value=0
  Constant1 : Constant  Value=0
  Data Store Write : DataStoreWrite  DataStoreName=messageTrigger2
  Data Store Write4 : DataStoreWrite  DataStoreName=removeMessageTrigger2
  wires:
  Constant/1 -> Data Store Write4/1
  Constant1/1 -> Data Store Write/1

== system platooning_with_csma_simulink/checks3/If Action Subsystem1 ==
  time : Inport
  velocity : Inport  Port=2
  position : Inport  Port=3
  Action Port : ActionPort  ActionType=then
  Constant : Constant
  Constant1 : Constant  Value=remove_trigger_time
  Data Store Read3 : DataStoreRead  DataStoreName=messageTrigger2
  Data Store Write : DataStoreWrite  DataStoreName=t2
  Data Store Write1 : DataStoreWrite  DataStoreName=messageTrigger2
  Data Store Write2 : DataStoreWrite  DataStoreName=v2
  Data Store Write3 : DataStoreWrite  DataStoreName=x2
  Data Store Write4 : DataStoreWrite  DataStoreName=removeMessageTrigger2
  Sum : Sum  Inputs=|++
  Sum1 : Sum  Inputs=|++
  wires:
  time/1 -> Sum1/1, Data Store Write/1
  position/1 -> Data Store Write3/1
  velocity/1 -> Data Store Write2/1
  Data Store Read3/1 -> Sum/1
  Constant/1 -> Sum/2
  Sum/1 -> Data Store Write1/1
  Sum1/1 -> Data Store Write4/1
  Constant1/1 -> Sum1/2

== system platooning_with_csma_simulink/checks4/If Action Subsystem ==
  Action Port : ActionPort  ActionType=then
  Constant : Constant  Value=0
  Constant1 : Constant  Value=0
  Data Store Write : DataStoreWrite  DataStoreName=messageTrigger3
  Data Store Write4 : DataStoreWrite  DataStoreName=removeMessageTrigger3
  wires:
  Constant/1 -> Data Store Write4/1
  Constant1/1 -> Data Store Write/1

== system platooning_with_csma_simulink/checks4/If Action Subsystem1 ==
  time : Inport
  velocity : Inport  Port=2
  position : Inport  Port=3
  Action Port : ActionPort  ActionType=then
  Constant : Constant
  Constant1 : Constant  Value=remove_trigger_time
  Data Store Read3 : DataStoreRead  DataStoreName=messageTrigger3
  Data Store Write : DataStoreWrite  DataStoreName=t3
  Data Store Write1 : DataStoreWrite  DataStoreName=messageTrigger3
  Data Store Write2 : DataStoreWrite  DataStoreName=v3
  Data Store Write3 : DataStoreWrite  DataStoreName=x3
  Data Store Write4 : DataStoreWrite  DataStoreName=removeMessageTrigger3
  Sum : Sum  Inputs=|++
  Sum1 : Sum  Inputs=|++
  wires:
  time/1 -> Sum1/1, Data Store Write/1
  position/1 -> Data Store Write3/1
  velocity/1 -> Data Store Write2/1
  Data Store Read3/1 -> Sum/1
  Constant/1 -> Sum/2
  Sum/1 -> Data Store Write1/1
  Sum1/1 -> Data Store Write4/1
  Constant1/1 -> Sum1/2
